simulink model "amc_simulator"  (R2024b)
settings: Solver=FixedStepDiscrete  StartTime=0.0  StopTime=2/50  RelTol=1e-3
InitFcn:
  | fac=8e6;
  | tac=1/(fac);
  | tcnt=tac;
model workspace (MAT data in the model file):
  cnt = Simulink.Parameter
  cnt.Value = 0
  cnt.Complexity = 'real'
  cnt.Dimensions = [1 1]
  cnt.DataType = 'uint8'
  cnt.Min = 0
  cnt.Max = 250
libraries: hdlsllib x2, dspsrcs4 x1
settings Model: DataTypeOverride=Off  Creator=angro  LastModifiedBy=Angel
settings SolverCC: AlgebraicLoopSolver=TrustRegion
settings DataIOCC: LimitDataPoints=on  SaveOutput=off  SaveTime=off
settings OptimizationCC: BlockReduction=off  ConditionallyExecuteInputs=off  DefaultParameterBehavior=Inlined  InheritOutputTypeSmallerThanSingle=on  ExpressionDepthLimit=2147483647  InitFltsAndDblsToZero=on  LifeSpan=inf
settings DebuggingCC: AlgebraicLoopMsg=error  MergeDetectMultiDrivingBlocksExec=none  SingleTaskRateTransMsg=error  FcnCallInpInsideContextMsg=warning  UnconnectedInputMsg=warning  UnconnectedOutputMsg=warning  UnconnectedLineMsg=warning  AllowSymbolicDim=off  StateNameClashWarn=warning  StrictBusMsg=ErrorOnBusTreatedAsVector  SFUnexpectedBacktrackingDiag=warning  SFNoUnconditionalDefaultTransitionDiag=warning  SFExecutionAtInitializationDiag=none  ArithmeticOperatorsInVariantConditions=warning
settings HardwareCC: ProdBitPerPointer=32  ProdBitPerSizeT=32  ProdBitPerPtrDiffT=32  ProdLargestAtomicFloat=None  ProdIntDivRoundTo=Undefined  ProdEndianess=Unspecified  ProdWordSize=32  ProdHWDeviceType=ASIC/FPGA->ASIC/FPGA  ProdEqTarget=off
settings ModelReferenceCC: EnableRefExpFcnMdlSchedulingChecks=on
settings SFSimCC: SimUseLocalCustomCode=off  SimParseCustomCode=off  CustomCodeUndefinedFunction=UseInterfaceOnly
settings RTWCC: PackageGeneratedCodeAndArtifacts=on  RTWUseLocalCustomCode=off  GPUComputeCapability=3.5
settings CodeAppCC: StateflowObjectComments=on
settings GRTTargetCC: TargetLangStandard=C89/C90 (ANSI)  CombineOutputUpdateFcns=off  GRTInterface=on
settings ConfigComp: CovScope=ReferencedModels  CovMetricSettings=dw  CovSaveCumulativeToWorkspaceVar=on  CovSaveSingleToWorkspaceVar=on  CovExternalEMLEnable=off  CovSFcnEnable=off

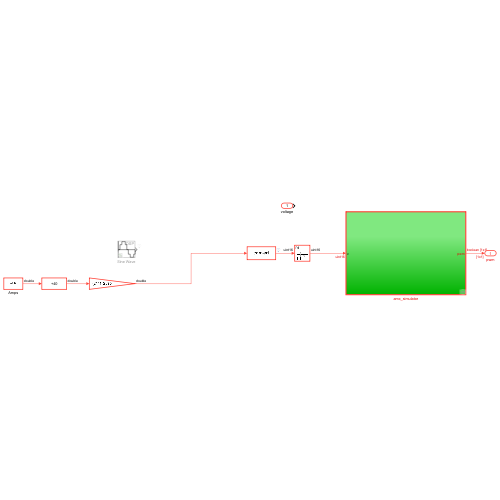
[thumbnail: Simulink's stored preview of the top-level diagram]
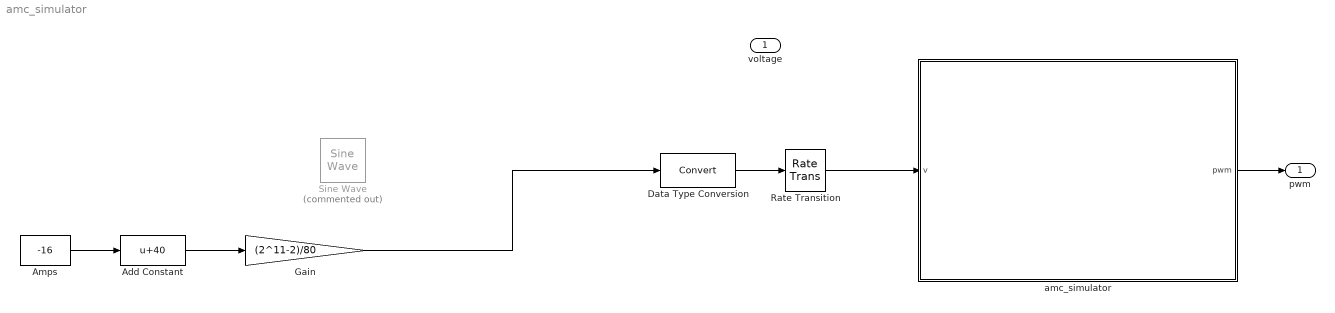
== system amc_simulator ==
  voltage : Inport
  Add Constant : Bias  Bias=40  SaturateOnIntegerOverflow=off
  Amps : Constant  Value=-16  SampleTime=-1
  Data Type Conversion : DataTypeConversion  OutMin=[0]  SaturateOnIntegerOverflow=off  RndMeth=Floor
  Gain : Gain  Gain=(2^11-2)/80
  Rate Transition : RateTransition
  Sine Wave : dspsrcs4/Sine Wave  Commented=on  Amplitude=4095/3  Frequency=50  Phase=0  SampleMode=Discrete  OutComplex=Real  CompMethod=Trigonometric fcn  TableSize=Speed  SampleTime=1/5000  SamplesPerFrame=1  ResetState=Restart at time zero  OutputFrames=off  dataType=single  wordLen=16  udDataType=sfix(16)  fracBitsMode=Best precision  numFracBits=15  OutDataTypeStr=single  LastOutDataTypeStr=single
  amc_simulator : Subsystem  TreatAsAtomicUnit=on  SystemSampleTime=1/30e6
  pwm : Outport
  wires:
  amc_simulator/1(pwm) -> pwm/1
  Data Type Conversion/1 -> Rate Transition/1
  Rate Transition/1 -> amc_simulator/1(v)
  Amps/1 -> Add Constant/1
  Add Constant/1 -> Gain/1
  Gain/1 -> Data Type Conversion/1

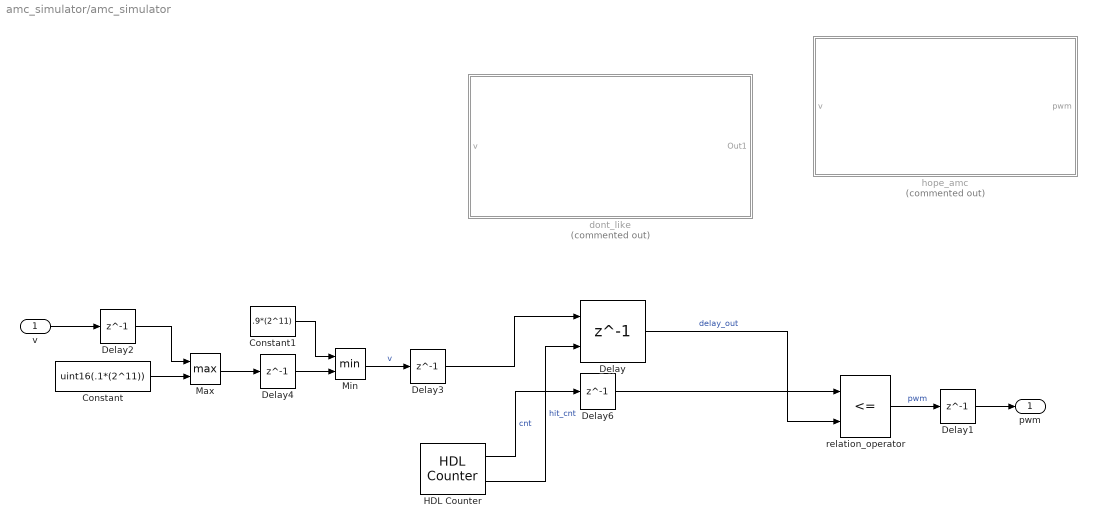
== system amc_simulator/amc_simulator ==
  v : Inport  OutMin=[0]  OutDataTypeStr=uint16
  Constant : Constant  Value=uint16(.1*(2^11))  SampleTime=-1
  Constant1 : Constant  Value=.9*(2^11)  VectorParams1D=off  OutDataTypeStr=uint16  SampleTime=-1
  Delay : Delay  DelayLength=1  InitialCondition=0  ShowEnablePort=on
      settings: InputPortMap=u0,e6
  Delay1 : Delay  DelayLength=1  InitialCondition=1
  Delay2 : Delay  DelayLength=1  InitialCondition=1
  Delay3 : Delay  DelayLength=1  InitialCondition=409
  Delay4 : Delay  DelayLength=1  InitialCondition=409
  Delay6 : Delay  DelayLength=1  InitialCondition=490
  HDL Counter : hdlsllib/Sources/HDL Counter  CountType=Count limited  CountInit=1  CountStep=1  CountMax=uint16((2^11)*1.1)  CountFromType=Initial value  CountFrom=1  CountResetPort=off  CountLoadPort=off  CountEnbPort=off  CountDirPort=off  CountHitOutputPort=on  CountDataType=Unsigned  CountWordLen=16  CountFracLen=0  CountSampTime=-1
  Max : MinMax  Function=max  Inputs=2
  Min : MinMax  Inputs=2
  dont_like : Subsystem  Commented=on
  hope_amc : Stateflow chart  Commented=on  TreatAsAtomicUnit=on
  relation_operator : RelationalOperator  Operator=<=  OutDataTypeStr=boolean  InputSameDT=off
  pwm : Outport
  wires:
  v/1 -> Delay2/1
  Constant1/1 -> Min/1
  Delay2/1 -> Max/1
  Constant/1 -> Max/2
  Delay3/1 -> Delay/1
  Delay4/1 -> Min/2
  Max/1 -> Delay4/1
  Min/1 -> Delay3/1  "v"
  HDL Counter/2 -> Delay/2  "hit_cnt"
  HDL Counter/1 -> Delay6/1  "cnt"
  Delay6/1 -> relation_operator/1
  Delay/1 -> relation_operator/2  "delay_out"
  relation_operator/1 -> Delay1/1  "pwm"
  Delay1/1 -> pwm/1

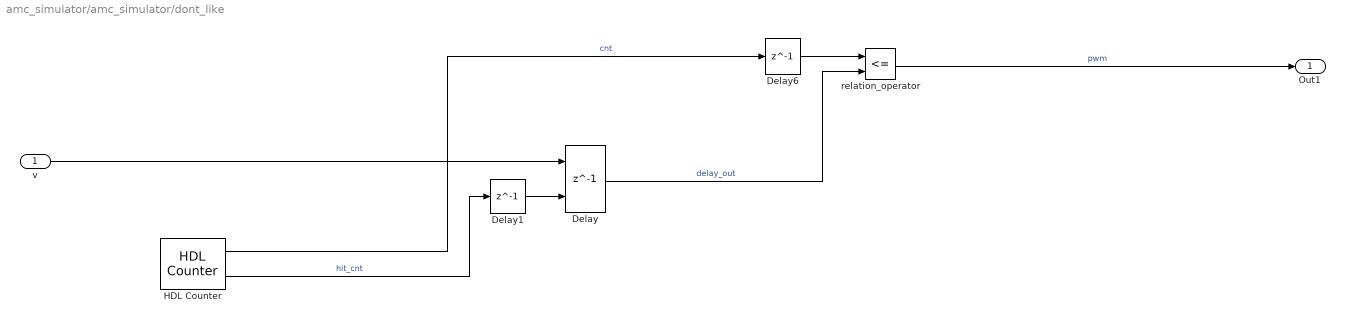
== system amc_simulator/amc_simulator/dont_like ==
  v : Inport
  Delay : Delay  DelayLength=1  InitialCondition=uint16(409)  ShowEnablePort=on
      settings: InputPortMap=u0,e6
  Delay1 : Delay  DelayLength=1  InitialCondition=1
  Delay6 : Delay  DelayLength=1  InitialCondition=490
  HDL Counter : hdlsllib/Sources/HDL Counter  CountType=Count limited  CountInit=1  CountStep=1  CountMax=4551+409  CountFromType=Initial value  CountFrom=1  CountResetPort=off  CountLoadPort=off  CountEnbPort=off  CountDirPort=off  CountHitOutputPort=on  CountDataType=Unsigned  CountWordLen=16  CountFracLen=0  CountSampTime=-1
  relation_operator : RelationalOperator  Operator=<=  OutDataTypeStr=boolean  InputSameDT=off
  Out1 : Outport
  wires:
  Delay6/1 -> relation_operator/1
  HDL Counter/2 -> Delay1/1  "hit_cnt"
  Delay1/1 -> Delay/2
  HDL Counter/1 -> Delay6/1  "cnt"
  Delay/1 -> relation_operator/2  "delay_out"
  relation_operator/1 -> Out1/1  "pwm"
  v/1 -> Delay/1

== stateflow chart amc_simulator/hope_amc ==
  state init
    en:
    v_reg = v;
    pwm=false;
    cnt=0;
  state inc_cnt
    en:
  (default) -> init
  (junction 28) -> init
  (junction 26) -> (junction 28)
  init -> inc_cnt
  (junction 23) -> inc_cnt
  inc_cnt -> (junction 26) [order 2] : [cnt>=uint16((2^12))]
  (junction 21) -> (junction 23)
  inc_cnt -> (junction 12) [order 1] : [cnt<uint16((2^12))]
  (junction 12) -> (junction 31) [order 2] : [(v_reg)<=cnt]{pwm=false}
  (junction 12) -> (junction 19) [order 1] : [(v_reg)>cnt]{pwm=true}
  (junction 31) -> (junction 33)
  (junction 19) -> (junction 21) : {cnt=cnt+1}
  (junction 33) -> (junction 19)
  data: v input; pwm output boolean; v_reg local uint16; cnt local uint16
